simulink model "plant"  (Simulink 7.7)
settings: Solver=ode45  StartTime=0.0  StopTime=10.0  RelTol=1e-3
values from neighbouring files (symbols this model uses):
  gamma = 0    [main.m]
  impulse = 0    [main.m]
  k_d = -k_p * 1    (= 0.005)    [main.m]
  k_i = k_p * .5    (= -0.0025)    [main.m]
  k_p = -.005    (= -0.005)    [main.m]
  noise = .1    (= 0.1)    [main.m]
  ref = 0    [main.m]
settings Model: Creator=Edward  LastModifiedBy=Edward

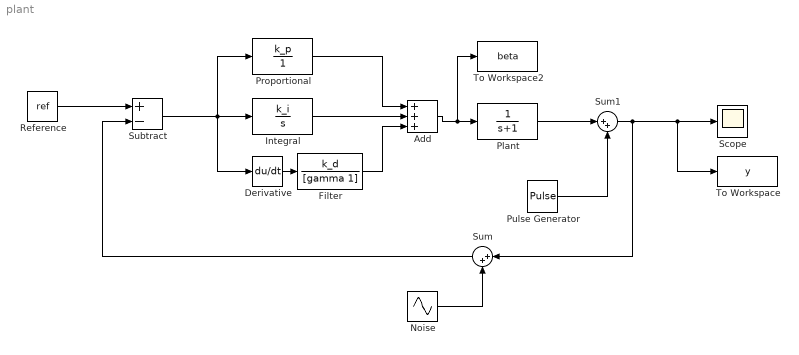
== system plant ==
  Add : Sum  Inputs=+++
  Derivative : Derivative
  Filter : TransferFcn  Numerator=k_d  Denominator=[gamma 1]
  Integral : TransferFcn  Numerator=k_i  Denominator=[1 0]
  Noise : Sin  Amplitude=noise  Frequency=377  SampleTime=0
  Plant : TransferFcn  Denominator=[1 1]
  Proportional : TransferFcn  Numerator=k_p  Denominator=1
  Pulse Generator : DiscretePulseGenerator  PulseType=Time based  Amplitude=impulse  Period=10  PulseWidth=5  PhaseDelay=1
  Reference : Constant  Value=ref
  Scope : Scope
  Subtract : Sum  Inputs=+-
  Sum : Sum  Inputs=|++
  Sum1 : Sum  Inputs=|++
  To Workspace : ToWorkspace  VariableName=y  SampleTime=-1  SaveFormat=Structure With Time
  To Workspace2 : ToWorkspace  VariableName=beta  SampleTime=-1  SaveFormat=Structure With Time
  wires:
  Reference/1 -> Subtract/1
  Subtract/1 -> Integral/1, Proportional/1, Derivative/1
  Proportional/1 -> Add/1
  Filter/1 -> Add/3
  Integral/1 -> Add/2
  Add/1 -> Plant/1, To Workspace2/1
  Plant/1 -> Sum1/1
  Sum1/1 -> Scope/1, To Workspace/1, Sum/1
  Noise/1 -> Sum/2
  Sum/1 -> Subtract/2
  Pulse Generator/1 -> Sum1/2
  Derivative/1 -> Filter/1
